simulink model "radiationForce_interp2"  (R2022a)
settings: Solver=ode3  StartTime=0.0  StopTime=30  FixedStep=0.01  RelTol=1e-3
undefined symbols (not defined in the file): aR2, aRInterp, B1_all, bR2, bRInterp, hydroCoeff, radA, radB, radC, tRamp, w_Wave, w_WaveIndx
libraries: simulink x2, cstblocks x2
settings Model: Creator=tdemonte  LastModifiedBy=tdemonte

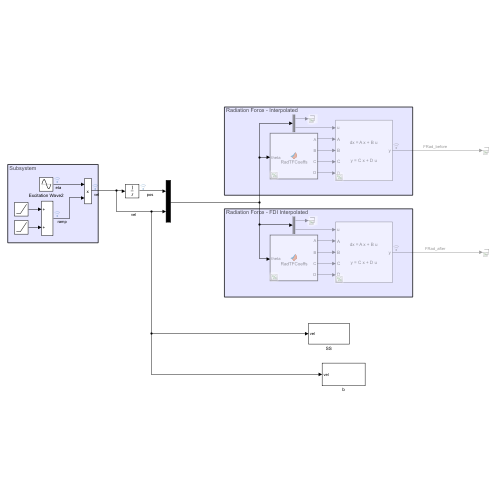
[thumbnail: Simulink's stored preview of the top-level diagram]
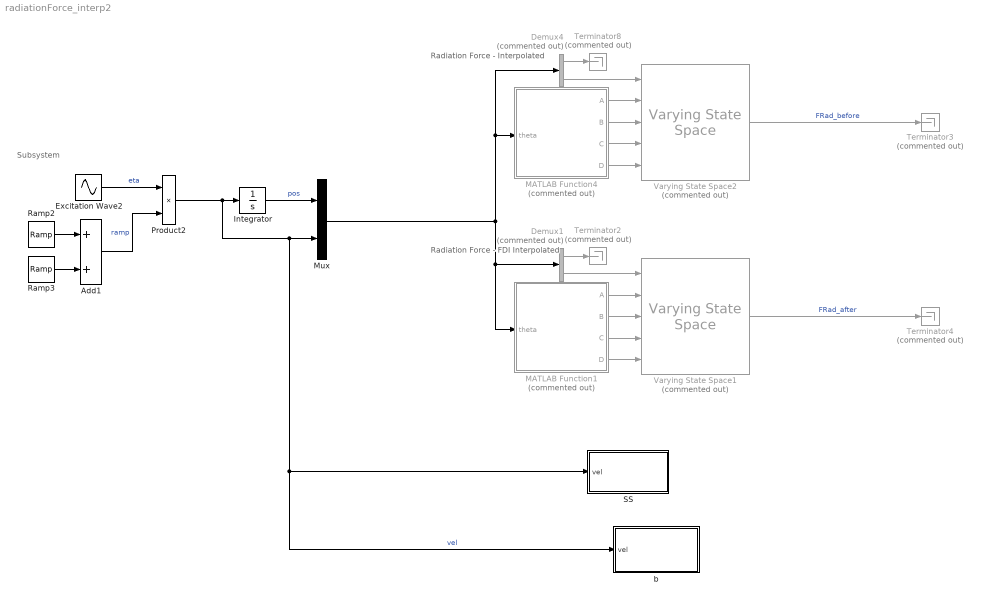
== system radiationForce_interp2 ==
  note: Radiation Force - Interpolated
  note: Radiation Force - FDI Interpolated
  note: Subsystem
  Add1 : Sum
  Demux1 : Demux  Commented=on  Outputs=2
  Demux4 : Demux  Commented=on  Outputs=2
  Excitation Wave2 : Sin  Frequency=w_Wave  SampleTime=0
  Integrator : Integrator
  MATLAB Function1 : MATLAB Function  Commented=on  TreatAsAtomicUnit=on
  MATLAB Function4 : MATLAB Function  Commented=on  TreatAsAtomicUnit=on
  Mux : Mux  Inputs=2
  Product2 : Product
  Ramp2 : simulink/Sources/Ramp  slope=1/tRamp  start=0  InitialOutput=0
  Ramp3 : simulink/Sources/Ramp  slope=-1/tRamp  start=tRamp  InitialOutput=0
  SS : Subsystem
  Terminator{2..4,8} (4 alike) : Terminator  Commented=on
  Varying State Space1 : cstblocks/Linear Parameter Varying/Varying State Space  Commented=on  x0=0  xNames=''  OutputX=off  OutputDX=off
  Varying State Space2 : cstblocks/Linear Parameter Varying/Varying State Space  Commented=on  x0=0  xNames=''  OutputX=off  OutputDX=off
  b : Subsystem
  wires:
  Demux4/2 -> Varying State Space2/1
  Mux/1 -> MATLAB Function1/1(theta), Demux1/1, Demux4/1, MATLAB Function4/1(theta)
  MATLAB Function4/2(B) -> Varying State Space2/3
  MATLAB Function4/1(A) -> Varying State Space2/2
  MATLAB Function4/4(D) -> Varying State Space2/5
  MATLAB Function4/3(C) -> Varying State Space2/4
  Varying State Space2/1 -> Terminator3/1  "FRad_before"
  Demux4/1 -> Terminator8/1
  Demux1/1 -> Terminator2/1
  Varying State Space1/1 -> Terminator4/1  "FRad_after"
  MATLAB Function1/3(C) -> Varying State Space1/4
  MATLAB Function1/4(D) -> Varying State Space1/5
  MATLAB Function1/1(A) -> Varying State Space1/2
  MATLAB Function1/2(B) -> Varying State Space1/3
  Demux1/2 -> Varying State Space1/1
  Excitation Wave2/1 -> Product2/1  "eta"
  Add1/1 -> Product2/2  "ramp"
  Ramp3/1 -> Add1/2
  Ramp2/1 -> Add1/1
  Product2/1 -> b/1(vel), SS/1(vel), Mux/2, Integrator/1  "vel"
  Integrator/1 -> Mux/1  "pos"

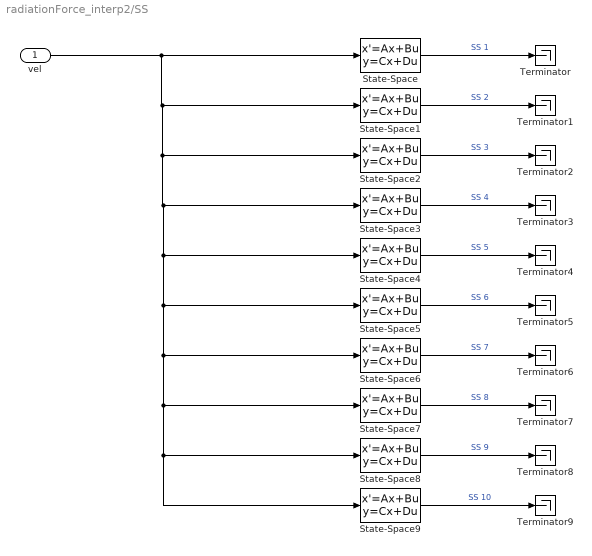
== system radiationForce_interp2/SS ==
  vel : Inport
  State-Space : StateSpace  A=radA{1}  B=radB{1}  C=radC{1}  D=0  InitialCondition=0
  State-Space1 : StateSpace  A=radA{2}  B=radB{2}  C=radC{2}  D=0  InitialCondition=0
  State-Space2 : StateSpace  A=radA{3}  B=radB{3}  C=radC{3}  D=0  InitialCondition=0
  State-Space3 : StateSpace  A=radA{4}  B=radB{4}  C=radC{4}  D=0  InitialCondition=0
  State-Space4 : StateSpace  A=radA{5}  B=radB{5}  C=radC{5}  D=0  InitialCondition=0
  State-Space5 : StateSpace  A=radA{6}  B=radB{6}  C=radC{6}  D=0  InitialCondition=0
  State-Space6 : StateSpace  A=radA{7}  B=radB{7}  C=radC{7}  D=0  InitialCondition=0
  State-Space7 : StateSpace  A=radA{8}  B=radB{8}  C=radC{8}  D=0  InitialCondition=0
  State-Space8 : StateSpace  A=radA{9}  B=radB{9}  C=radC{9}  D=0  InitialCondition=0
  State-Space9 : StateSpace  A=radA{10}  B=radB{10}  C=radC{10}  D=0  InitialCondition=0
  Terminator{,1..9} (10 alike) : Terminator
  wires:
  State-Space/1 -> Terminator/1  "SS 1"
  State-Space1/1 -> Terminator1/1  "SS 2"
  State-Space2/1 -> Terminator2/1  "SS 3"
  State-Space3/1 -> Terminator3/1  "SS 4"
  State-Space4/1 -> Terminator4/1  "SS 5"
  State-Space5/1 -> Terminator5/1  "SS 6"
  State-Space6/1 -> Terminator6/1  "SS 7"
  State-Space7/1 -> Terminator7/1  "SS 8"
  State-Space8/1 -> Terminator8/1  "SS 9"
  vel/1 -> State-Space9/1, State-Space8/1, State-Space7/1, State-Space6/1, State-Space5/1, State-Space4/1, State-Space3/1, State-Space2/1, State-Space1/1, State-Space/1
  State-Space9/1 -> Terminator9/1  "SS 10"

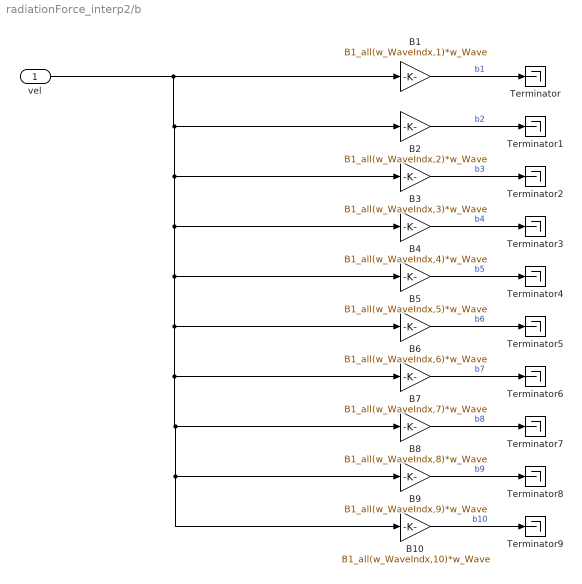
== system radiationForce_interp2/b ==
  vel : Inport
  B1 : Gain  Gain=B1_all(w_WaveIndx,1)*w_Wave
  B10 : Gain  Gain=B1_all(w_WaveIndx,10)*w_Wave
  B2 : Gain  Gain=B1_all(w_WaveIndx,2)*w_Wave
  B3 : Gain  Gain=B1_all(w_WaveIndx,3)*w_Wave
  B4 : Gain  Gain=B1_all(w_WaveIndx,4)*w_Wave
  B5 : Gain  Gain=B1_all(w_WaveIndx,5)*w_Wave
  B6 : Gain  Gain=B1_all(w_WaveIndx,6)*w_Wave
  B7 : Gain  Gain=B1_all(w_WaveIndx,7)*w_Wave
  B8 : Gain  Gain=B1_all(w_WaveIndx,8)*w_Wave
  B9 : Gain  Gain=B1_all(w_WaveIndx,9)*w_Wave
  Terminator{,1..9} (10 alike) : Terminator
  wires:
  B1/1 -> Terminator/1  "b1"
  B2/1 -> Terminator1/1  "b2"
  B3/1 -> Terminator2/1  "b3"
  B4/1 -> Terminator3/1  "b4"
  B5/1 -> Terminator4/1  "b5"
  B6/1 -> Terminator5/1  "b6"
  B7/1 -> Terminator6/1  "b7"
  B8/1 -> Terminator7/1  "b8"
  B9/1 -> Terminator8/1  "b9"
  B10/1 -> Terminator9/1  "b10"
  vel/1 -> B10/1, B9/1, B8/1, B7/1, B6/1, B5/1, B4/1, B3/1, B2/1, B1/1

== matlab function radiationForce_interp2/MATLAB Function1 ==
  data: theta input; A output size=[6 6]; B output size=[6 1]; hydroCoeff parameter; C output size=[1 6]; D output size=1; aR2 parameter; bR2 parameter
function [A,B,C,D] = RadTFCoeffs(theta, hydroCoeff, aR2, bR2)
% This function extracts the coefficients of the Radiation Transfer
% Function based on previously fitted data between discretized thetas. 

% Inputs: 
% theta0      = current states condition
% hydrovCoeff = time-variable hydrodynamic coefficients
% thetaN      = pitch angle index

% Outputs: 
% bR    = numerator 
% aR    = denominator 

% States: 
theta1  = theta(1); % (1) theta:  pitch angle response
% theta2  = theta(2); % (2) thetaD: pitch angle velocity


% Find the index for the discretized theta 
theta1N = wrapToPi(theta1); 

if abs(rad2deg(theta1N)) >= 95
    theta1N = pi - abs(theta1N); 
end 

thetaN = find(deg2rad(hydroCoeff.theta) > abs(theta1N),1); 
% % Get transfer function coefficients depending on the discretized angle. 
aR       = zeros(1,7); 
bR       = zeros(1,7);
% 
aR(:)    = aR2(thetaN,:);
bR(:)    = bR2(thetaN,:);
% 
n = nnz(aR);
% 
% if n<7
%     aR(1) = 0;
% end
% if n<6
%     aR(2) = 0;
% end
% % Get transfer function coefficients depending on the discretized angle. 
A       = zeros(6,6); 
B       = zeros(6,1); 
C       = zeros(1,6); 
D       = 0; 

[A(end-n+2:end,end-n+2:end), B(end-n+2:end,1), C(1,end-n+2:end), D(1)] = tf2ss(-bR,-aR);

% B(end-n+2)  = 1; 
% A(end-n+2,end-n+2) = 1; 
% A(1:end-n+1,1:end-n+1) = 0; 
% [A(end-n+2:end,end-n+2:end), B(end-n+2:end,1), C(1,end-n+2:end), D(1)] = tf2ss(-bR,-aR);

== matlab function radiationForce_interp2/MATLAB Function4 ==
  data: theta input; A output size=[6 6]; B output size=[6 1]; hydroCoeff parameter; C output size=[1 6]; D output size=1; aRInterp parameter; bRInterp parameter
function [A,B,C,D] = RadTFCoeffs(theta, hydroCoeff, aRInterp, bRInterp)
% This function extracts the coefficients of the Radiation Transfer
% Function based on previously fitted data between discretized thetas. 

% Inputs: 
% theta0      = current states condition
% hydrovCoeff = time-variable hydrodynamic coefficients
% thetaN      = pitch angle index

% Outputs: 
% bR    = numerator 
% aR    = denominator 

% States: 
theta1  = theta(1); % (1) theta:  pitch angle response
% theta2  = theta(2); % (2) thetaD: pitch angle velocity


% Find the index for the discretized theta 
theta1N = wrapToPi(theta1); 

if abs(rad2deg(theta1N)) >= 90 
    theta1N = pi - abs(theta1N); 
end 

thetaN = find(deg2rad(hydroCoeff.fineTheta) > abs(theta1N),1)-1; 
% % Get transfer function coefficients depending on the discretized angle. 
aR       = zeros(1,7); 
bR       = zeros(1,7);

aR(1,:)    = aRInterp(:,thetaN);
bR(1,:)    = bRInterp(:,thetaN);

n = nnz(aR);
% % Get transfer function coefficients depending on the discretized angle. 
A       = zeros(6,6); 
B       = zeros(6,1); 
C       = zeros(1,6); 
D       = 0; 

[A(:,:), B(:,1), C(1,:), D(1)] = tf2ss(bR,aR);
